simulink model "modelisation_simu"  (R2024b)
settings: Solver=VariableStepAuto  StartTime=0.0  StopTime=10.0  RelTol=1e-3
values from neighbouring files (symbols this model uses):
  den1 = [5.0139 41.3247 69.0255] * 1.2    [generate_data.m]
  den2 = [15.0293 123.8716 206.9052]    [generate_data.m]
  den3 = [15.9337 131.3254 219.3554]    [generate_data.m]
  den4 = [9.3766 77.2822 129.0860]    [generate_data.m]
  num1 = 141.6180    (= 141.618)    [generate_data.m]
  num2 = 245.1882    [generate_data.m]
  num3 = 252.4573    [generate_data.m]
  num4 = 193.6660    (= 193.666)    [generate_data.m]
settings Model: Creator=elasr  LastModifiedBy=elasr

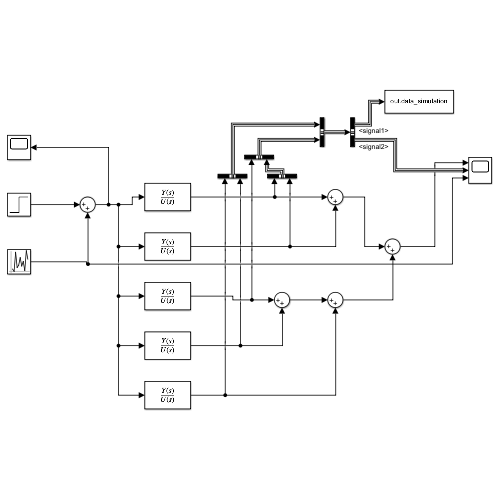
[thumbnail: Simulink's stored preview of the top-level diagram]
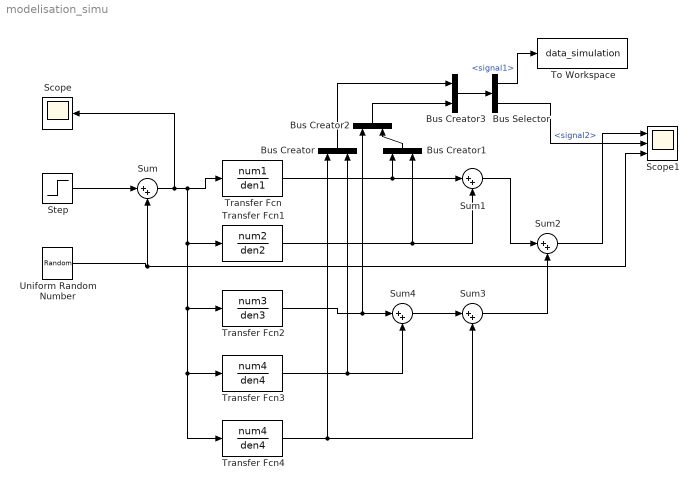
== system modelisation_simu ==
  Bus Creator{,1..3} (4 alike) : BusCreator  Inputs=2
  Bus Selector : BusSelector  OutputSignals=signal1,signal2
  Scope : Scope
  Scope1 : Scope  NumInputPorts=3
  Step : Step  SampleTime=0
  Sum{,1..4} (5 alike) : Sum  Inputs=|++
  To Workspace : ToWorkspace  VariableName=data_simulation  SampleTime=-1
  Transfer Fcn : TransferFcn  Numerator=num1  Denominator=den1
  Transfer Fcn1 : TransferFcn  Numerator=num2  Denominator=den2
  Transfer Fcn2 : TransferFcn  Numerator=num3  Denominator=den3
  Transfer Fcn3 : TransferFcn  Numerator=num4  Denominator=den4
  Transfer Fcn4 : TransferFcn  Numerator=num4  Denominator=den4
  Uniform Random Number : UniformRandomNumber  SampleTime=0.1
  wires:
  Step/1 -> Sum/1
  Sum/1 -> Scope/1, Transfer Fcn/1, Transfer Fcn1/1, Transfer Fcn2/1, Transfer Fcn4/1, Transfer Fcn3/1
  Transfer Fcn/1 -> Bus Creator1/1, Sum1/1
  Transfer Fcn1/1 -> Bus Creator1/2, Sum1/2
  Sum1/1 -> Sum2/1
  Sum2/1 -> Scope1/1
  Sum3/1 -> Sum2/2
  Sum4/1 -> Sum3/1
  Transfer Fcn2/1 -> Bus Creator2/1, Sum4/1
  Transfer Fcn3/1 -> Sum4/2, Bus Creator/2
  Transfer Fcn4/1 -> Sum3/2, Bus Creator/1
  Uniform Random Number/1 -> Sum/2, Scope1/3
  Bus Creator1/1 -> Bus Creator2/2
  Bus Creator2/1 -> Bus Creator3/2
  Bus Creator/1 -> Bus Creator3/1
  Bus Creator3/1 -> Bus Selector/1
  Bus Selector/1 -> To Workspace/1  "<signal1>"
  Bus Selector/2 -> Scope1/2  "<signal2>"
